simulink model "TestVehicule"  (R2019b)
settings: Solver=VariableStepAuto  StartTime=0.0  StopTime=10.0  RelTol=1e-3
values from neighbouring files (symbols this model uses):
  ess_coulombic_eff = 0.99    [Batteries.m]
  ess_max_ah_cap = 28    [Batteries.m]
  ess_module_number = 20    [Batteries.m]
  ess_r = [0.01266 0.00685	0.00644	0.00599	0.00587	0.00575	0.00568	0.00581	0.00623	0.00667  0.00635]    [Batteries.m]
  ess_soc = [0:.1:1]    [Batteries.m]
  ess_tau = 0.1    [Batteries.m]
  ess_voc = [12.5 12.8 13.1 13.3 13.4 13.4 13.5 13.6 13.7 13.9 14.2]    [Batteries.m]
  gb_eff = [0.98 0.98 0.98 0.98 0.98]    [BoiteVitesse.m]
  gb_no = [1 2 3 4 5]    [BoiteVitesse.m]
  gb_ratio = [10 8 5 4 2]    [BoiteVitesse.m]
  mc_eff_map = 0.01*[ 20	20	20	20	20	20	20	20	20	20	20	20	20	20	20	20	20	20	20	20	20 ... (first row only)    [MachineElectrique.m]
  mc_inertia = 0.0226    [MachineElectrique.m]
  mc_map_spd = [0 500 1000 1500 2000 2500 3000 4000 5000 6000 7000]*(2*pi)/60    [MachineElectrique.m]
  mc_max_trq = [512 508.1 504.2 500.3 496.3	492.4 488.5 480.7 472.8 465 0]    *4.448/3.281/12    [MachineElectrique.m]
  mc_min_trq = -1*[512 508.1 504.2 500.3 496.3	492.4 488.5 480.7 472.8 465 0]    *4.448/3.281/12    [MachineElectrique.m]
  veh_A = 0.15    [Vehicule.m]
  veh_B = 4.87e-04    (= 0.000487)    [Vehicule.m]
  veh_C = 1.18e-06    [Vehicule.m]
  veh_cx = 0.35    [Vehicule.m]
  veh_gravity = 9.81    [Vehicule.m]
  veh_mass = 1500    [Vehicule.m]
  veh_r = 0.29    [Vehicule.m]
  veh_rho = 1.2    [Vehicule.m]
  veh_rr_alpha = -0.4745    [Vehicule.m]
  veh_rr_beta = 0.9552    [Vehicule.m]
  veh_S = 3    [Vehicule.m]
  veh_wpressure = 240    [Vehicule.m]
settings Model: Creator=szhang6_  LastModifiedBy=szhang6_
settings DataIOCC: ReturnWorkspaceOutputs=off

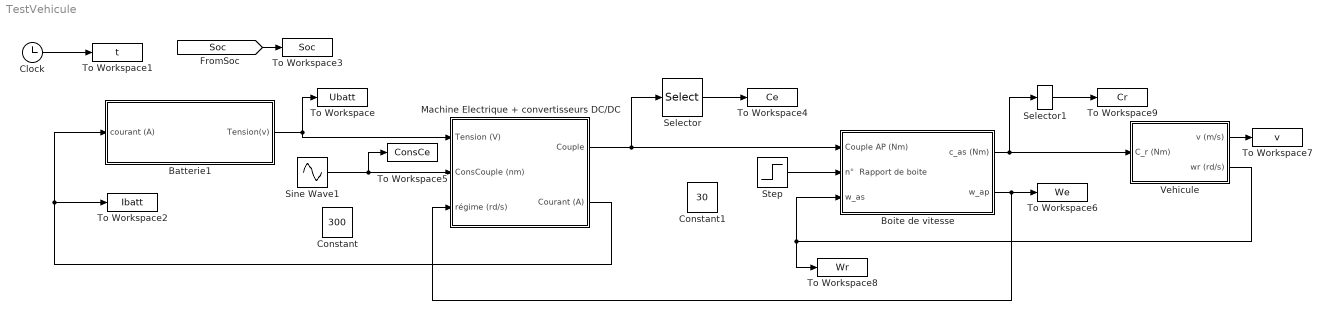
== system TestVehicule ==
  Batterie1 : Subsystem
  Boite de vitesse : Subsystem
  Clock : Clock
  Constant : Constant  Value=300
  Constant1 : Constant  Value=30
  Machine Electrique + convertisseurs DC/DC : Subsystem
  Selector : Selector  InputPortWidth=2  IndexOptions=Index vector (dialog)  Indices=1  OutputSizes=1
  Selector1 : Selector  InputPortWidth=2  IndexOptions=Index vector (dialog)  Indices=1  OutputSizes=1
  Sine Wave1 : Sin  SampleTime=0
  Step : Step  Time=5  Before=2  After=3  SampleTime=0
  To Workspace : ToWorkspace  VariableName=Ubatt  SampleTime=-1
  To Workspace1 : ToWorkspace  VariableName=t  SampleTime=-1
  To Workspace2 : ToWorkspace  VariableName=Ibatt  SampleTime=-1
  To Workspace3 : ToWorkspace  VariableName=Soc  SampleTime=-1
  To Workspace4 : ToWorkspace  VariableName=Ce  SampleTime=-1
  To Workspace5 : ToWorkspace  VariableName=ConsCe  SampleTime=-1
  To Workspace6 : ToWorkspace  VariableName=We  SampleTime=-1
  To Workspace7 : ToWorkspace  VariableName=v  SampleTime=-1
  To Workspace8 : ToWorkspace  VariableName=Wr  SampleTime=-1
  To Workspace9 : ToWorkspace  VariableName=Cr  SampleTime=-1
  Vehicule : Subsystem
  wires:
  Step/1 -> Boite de vitesse/2(n°  Rapport de boite)
  Vehicule/2(wr (rd/s)) -> Boite de vitesse/3(w_as), To Workspace8/1
  Machine Electrique + convertisseurs DC/DC/1(Couple) -> Boite de vitesse/1(Couple AP (Nm)), Selector/1
  Machine Electrique + convertisseurs DC/DC/2(Courant (A)) -> Batterie1/1(courant (A)), To Workspace2/1
  [Soc] -> To Workspace3/1
  Batterie1/1(Tension(v)) -> Machine Electrique + convertisseurs DC/DC/1(Tension (V)), To Workspace/1
  Sine Wave1/1 -> To Workspace5/1, Machine Electrique + convertisseurs DC/DC/2(ConsCouple (nm))
  Selector/1 -> To Workspace4/1
  Selector1/1 -> To Workspace9/1
  Clock/1 -> To Workspace1/1
  Boite de vitesse/1(c_as (Nm)) -> Vehicule/1(C_r (Nm)), Selector1/1
  Vehicule/1(v (m/s)) -> To Workspace7/1
  Boite de vitesse/2(w_ap) -> To Workspace6/1, Machine Electrique + convertisseurs DC/DC/3(régime (rd/s))

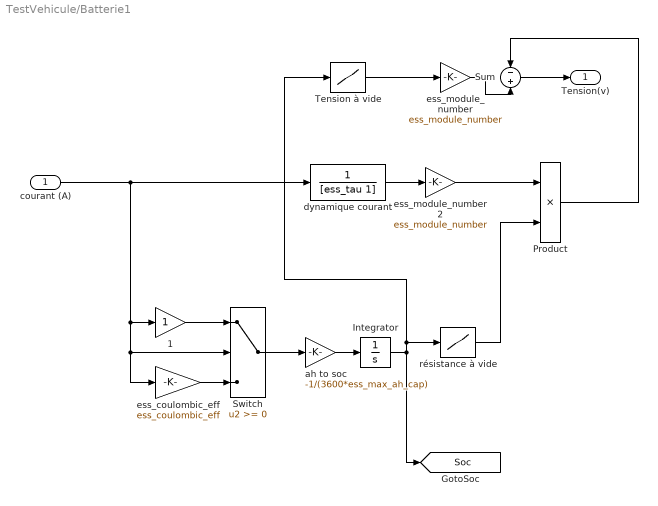
== system TestVehicule/Batterie1 ==
  courant (A) : Inport
  1 : Gain
  Integrator : Integrator
  Product : Product  Inputs=**
  Sum : Sum  Inputs=-+
  Switch : Switch
  Tension à vide : Lookup  InputValues=ess_soc  Table=ess_voc
  "ah to soc " : Gain  Gain=-1/(3600*ess_max_ah_cap)
  dynamique courant : TransferFcn  Denominator=[ess_tau 1]
  "ess_coulombic_eff " : Gain  Gain=ess_coulombic_eff
  "ess_module_number " : Gain  Gain=ess_module_number
  ess_module_number 2 : Gain  Gain=ess_module_number
  résistance à vide : Lookup  InputValues=ess_soc  Table=ess_r
  Tension(v) : Outport
  tag scope: Soc=global
  wires:
  courant (A)/1 -> dynamique courant/1, "ess_coulombic_eff "/1, Switch/2, 1/1
  1/1 -> Switch/1
  "ess_coulombic_eff "/1 -> Switch/3
  Switch/1 -> "ah to soc "/1
  "ah to soc "/1 -> Integrator/1
  dynamique courant/1 -> ess_module_number 2/1
  Integrator/1 -> [Soc], Tension à vide/1, résistance à vide/1
  ess_module_number 2/1 -> Product/1
  résistance à vide/1 -> Product/2
  Product/1 -> Sum/1
  Sum/1 -> Tension(v)/1
  Tension à vide/1 -> "ess_module_number "/1
  "ess_module_number "/1 -> Sum/2

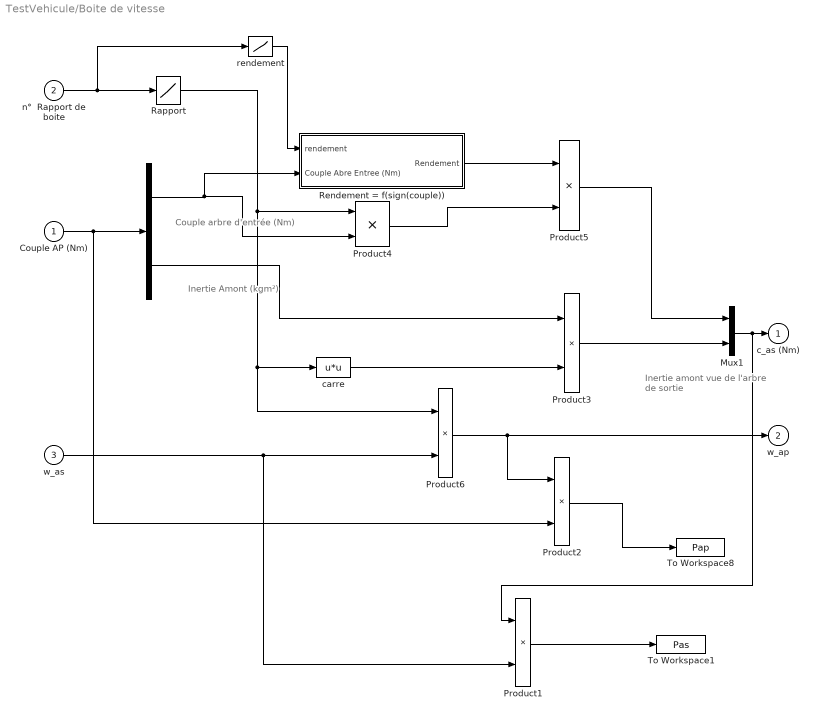
== system TestVehicule/Boite de vitesse ==
  note: Inertie
      |  Amont
      | (kgm²)
  note: Couple arbre
      |  d'entrée
      | (Nm)
  note: Inertie amont
      |  vue de
      |  l'arbre de sortie
  Couple AP (Nm) : Inport
  n°  Rapport de boite : Inport  Port=2
  w_as : Inport  Port=3
  " " : Demux  Outputs=2
  Mux1 : Mux  Inputs=2
  Product{1..2,4..6} (5 alike) : Product  SaturateOnIntegerOverflow=on  RndMeth=Zero  InputSameDT=on  OutDataTypeStr=Inherit: Same as first input
  Product3 : Product  Inputs=**  SaturateOnIntegerOverflow=on  RndMeth=Zero  InputSameDT=on  OutDataTypeStr=Inherit: Same as first input
  Rapport : Lookup  InputValues=gb_no  Table=gb_ratio
  Rendement = f(sign(couple)) : Subsystem
  To Workspace1 : ToWorkspace  VariableName=Pas  SampleTime=-1
  To Workspace8 : ToWorkspace  VariableName=Pap  SampleTime=-1
  carre : Fcn  Expr=u*u
  rendement : Lookup  InputValues=gb_no  Table=gb_eff
  c_as (Nm) : Outport  InitialOutput=0
  w_ap : Outport  Port=2  InitialOutput=0
  wires:
  " "/1 -> Product4/2, Rendement = f(sign(couple))/2(Couple Abre Entree (Nm))
  Mux1/1 -> Product1/1, c_as (Nm)/1
  Couple AP (Nm)/1 -> Product2/2, " "/1
  " "/2 -> Product3/1
  Product3/1 -> Mux1/2
  n°  Rapport de boite/1 -> rendement/1, Rapport/1
  rendement/1 -> Rendement = f(sign(couple))/1(rendement)
  Rapport/1 -> carre/1, Product6/1, Product4/1
  Rendement = f(sign(couple))/1(Rendement) -> Product5/1
  Product4/1 -> Product5/2
  Product5/1 -> Mux1/1
  w_as/1 -> Product1/2, Product6/2
  carre/1 -> Product3/2
  Product6/1 -> Product2/1, w_ap/1
  Product2/1 -> To Workspace8/1
  Product1/1 -> To Workspace1/1

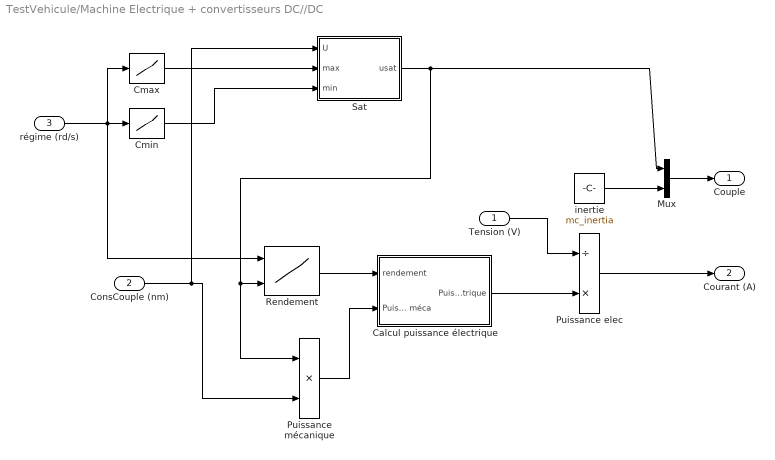
== system TestVehicule/Machine Electrique + convertisseurs DC//DC ==
  Tension (V) : Inport
  ConsCouple (nm) : Inport  Port=2
  régime (rd/s) : Inport  Port=3
  Calcul puissance électrique : Subsystem
  Cmax : Lookup  InputValues=mc_map_spd  Table=mc_max_trq
  Cmin : Lookup  InputValues=mc_map_spd  Table=mc_min_trq
  Mux : Mux  Inputs=2
  "Puissance elec " : Product  Inputs=/*
  Puissance mécanique : Product  Inputs=**
  Rendement : Lookup2D  RowIndex=mc_map_spd  ColumnIndex=mc_map_trq  Table=mc_eff_map  SaturateOnIntegerOverflow=on  InputSameDT=on
  Sat : Subsystem
  inertie : Constant  Value=mc_inertia
  Couple : Outport
  Courant (A) : Outport  Port=2
  wires:
  régime (rd/s)/1 -> Rendement/1, Cmax/1, Cmin/1
  Rendement/1 -> Calcul puissance électrique/1(rendement)
  Mux/1 -> Couple/1
  Calcul puissance électrique/1(Puissance électrique) -> "Puissance elec "/2
  "Puissance elec "/1 -> Courant (A)/1
  Puissance mécanique/1 -> Calcul puissance électrique/2(Puissance méca)
  inertie/1 -> Mux/2
  ConsCouple (nm)/1 -> Sat/1(U), Puissance mécanique/2
  Cmax/1 -> Sat/2(max)
  Cmin/1 -> Sat/3(min)
  Tension (V)/1 -> "Puissance elec "/1
  Sat/1(usat) -> Rendement/2, Puissance mécanique/1, Mux/1

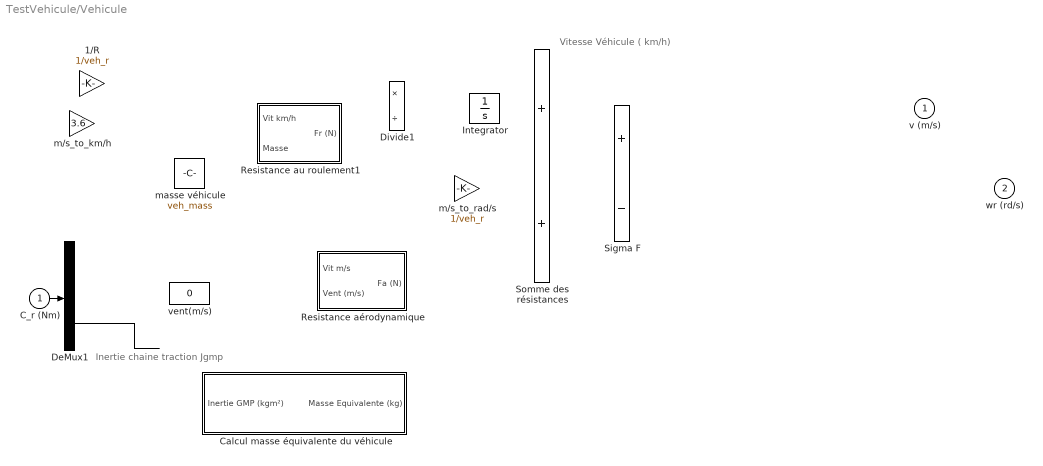
== system TestVehicule/Vehicule ==
  note: Inertie chaine traction
      | Jgmp
  note: Vitesse Véhicule ( km/h)
  C_r (Nm) : Inport
  1/R : Gain  Gain=1/veh_r  SaturateOnIntegerOverflow=on  OutDataTypeStr=Inherit: Same as input  ParamDataTypeStr=Inherit: Same as input
  Calcul masse équivalente du véhicule : Subsystem
  DeMux1 : Demux  Outputs=2
  Divide1 : Product  Inputs=*/
  Integrator : Integrator  InitialCondition=0.0001  LimitOutput=on  LowerSaturationLimit=0
  Resistance au roulement1 : Subsystem
  Resistance aérodynamique : Subsystem
  Sigma F : Sum  Inputs=+-  SaturateOnIntegerOverflow=on  InputSameDT=on  OutDataTypeStr=Inherit: Same as first input
  Somme des résistances : Sum  SaturateOnIntegerOverflow=on  InputSameDT=on  OutDataTypeStr=Inherit: Same as first input
  m/s_to_km/h : Gain  Gain=3.6  SaturateOnIntegerOverflow=on  OutDataTypeStr=Inherit: Same as input  ParamDataTypeStr=Inherit: Same as input
  m/s_to_rad/s : Gain  Gain=1/veh_r  SaturateOnIntegerOverflow=on  OutDataTypeStr=Inherit: Same as input  ParamDataTypeStr=Inherit: Same as input
  masse véhicule : Constant  Value=veh_mass
  vent(m/s) : Constant  Value=0
  v (m/s) : Outport  InitialOutput=0
  wr (rd/s) : Outport  Port=2  InitialOutput=0
  wires:
  C_r (Nm)/1 -> DeMux1/1
  DeMux1/2 -> ?

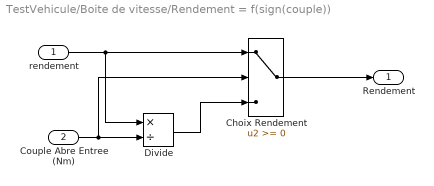
== system TestVehicule/Boite de vitesse/Rendement = f(sign(couple)) ==
  rendement : Inport
  Couple Abre Entree (Nm) : Inport  Port=2
  Choix Rendement : Switch  SaturateOnIntegerOverflow=on  InputSameDT=on
  Divide : Product  Inputs=*/
  Rendement : Outport  InitialOutput=0
  wires:
  rendement/1 -> Divide/1, Choix Rendement/1
  Choix Rendement/1 -> Rendement/1
  Couple Abre Entree (Nm)/1 -> Divide/2, Choix Rendement/2
  Divide/1 -> Choix Rendement/3

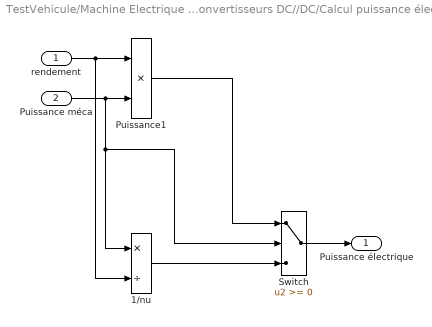
== system TestVehicule/Machine Electrique + convertisseurs DC//DC/Calcul puissance électrique ==
  rendement : Inport
  Puissance méca : Inport  Port=2
  1/nu : Product  Inputs=*/
  Puissance1 : Product  Inputs=**
  Switch : Switch
  Puissance électrique : Outport
  wires:
  rendement/1 -> 1/nu/2, Puissance1/1
  Puissance1/1 -> Switch/1
  1/nu/1 -> Switch/3
  Switch/1 -> Puissance électrique/1
  Puissance méca/1 -> 1/nu/1, Switch/2, Puissance1/2

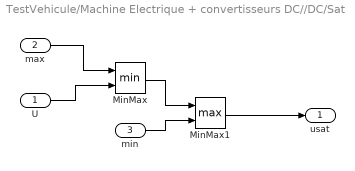
== system TestVehicule/Machine Electrique + convertisseurs DC//DC/Sat ==
  U : Inport
  max : Inport  Port=2
  min : Inport  Port=3
  MinMax : MinMax  Inputs=2
  MinMax1 : MinMax  Function=max  Inputs=2
  usat : Outport
  wires:
  max/1 -> MinMax/1
  U/1 -> MinMax/2
  MinMax/1 -> MinMax1/1
  min/1 -> MinMax1/2
  MinMax1/1 -> usat/1

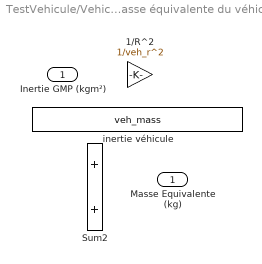
== system TestVehicule/Vehicule/Calcul masse équivalente du véhicule ==
  Inertie GMP (kgm²) : Inport
  1/R^2 : Gain  Gain=1/veh_r^2  SaturateOnIntegerOverflow=on  OutDataTypeStr=Inherit: Same as input  ParamDataTypeStr=Inherit: Same as input
  Sum2 : Sum  SaturateOnIntegerOverflow=on  InputSameDT=on  OutDataTypeStr=Inherit: Same as first input
  inertie véhicule : Constant  Value=veh_mass
  Masse Equivalente (kg) : Outport  InitialOutput=0

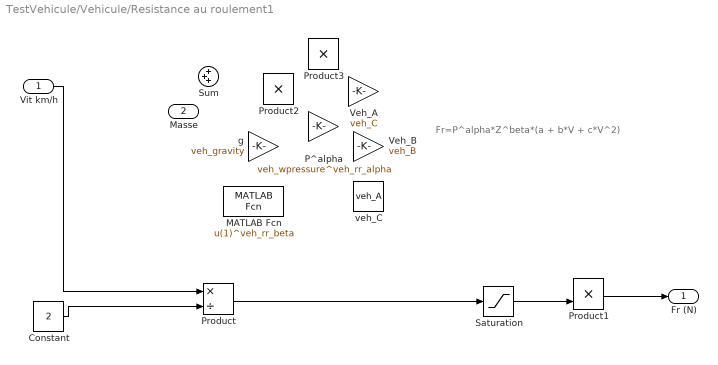
== system TestVehicule/Vehicule/Resistance au roulement1 ==
  note: Fr=P^alpha*Z^beta*(a + b*V + c*V^2)
  Vit km/h : Inport
  Masse : Inport  Port=2
  Constant : Constant  Value=2
  MATLAB Fcn : MATLABFcn  MATLABFcn=u(1)^veh_rr_beta
  "P^alpha " : Gain  Gain=veh_wpressure^veh_rr_alpha
  Product : Product  Inputs=*/  SaturateOnIntegerOverflow=on  InputSameDT=on  OutDataTypeStr=Inherit: Same as first input
  Product1 : Product  Inputs=**  SaturateOnIntegerOverflow=on  InputSameDT=on  OutDataTypeStr=Inherit: Same as first input
  Product2 : Product  Inputs=**  SaturateOnIntegerOverflow=on  InputSameDT=on  OutDataTypeStr=Inherit: Same as first input
  Product3 : Product  Inputs=**  SaturateOnIntegerOverflow=on  InputSameDT=on  OutDataTypeStr=Inherit: Same as first input
  Saturation : Saturate  UpperLimit=1  LowerLimit=0
  Sum : Sum  Inputs=+++
  Veh_A : Gain  Gain=veh_C
  Veh_B : Gain  Gain=veh_B
  g : Gain  Gain=veh_gravity
  veh_C : Constant  Value=veh_A
  Fr (N) : Outport  InitialOutput=0
  wires:
  Product1/1 -> Fr (N)/1
  Saturation/1 -> Product1/2
  Product/1 -> Saturation/1
  Constant/1 -> Product/2
  Vit km/h/1 -> Product/1
  ? -> Product1/1  "connecter Fr ici"

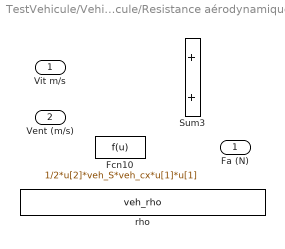
== system TestVehicule/Vehicule/Resistance aérodynamique ==
  Vit m/s : Inport
  Vent (m/s) : Inport  Port=2
  Fcn10 : Fcn  Expr=1/2*u[2]*veh_S*veh_cx*u[1]*u[1]
  Sum3 : Sum  SaturateOnIntegerOverflow=on  InputSameDT=on  OutDataTypeStr=Inherit: Same as first input
  rho : Constant  Value=veh_rho
  Fa (N) : Outport  InitialOutput=0
